simulink model "UDE"  (R2020b)
settings: Solver=VariableStepAuto  StartTime=0.0  StopTime=10.0  RelTol=1e-3
settings Model: Creator=ashya  LastModifiedBy=ashya

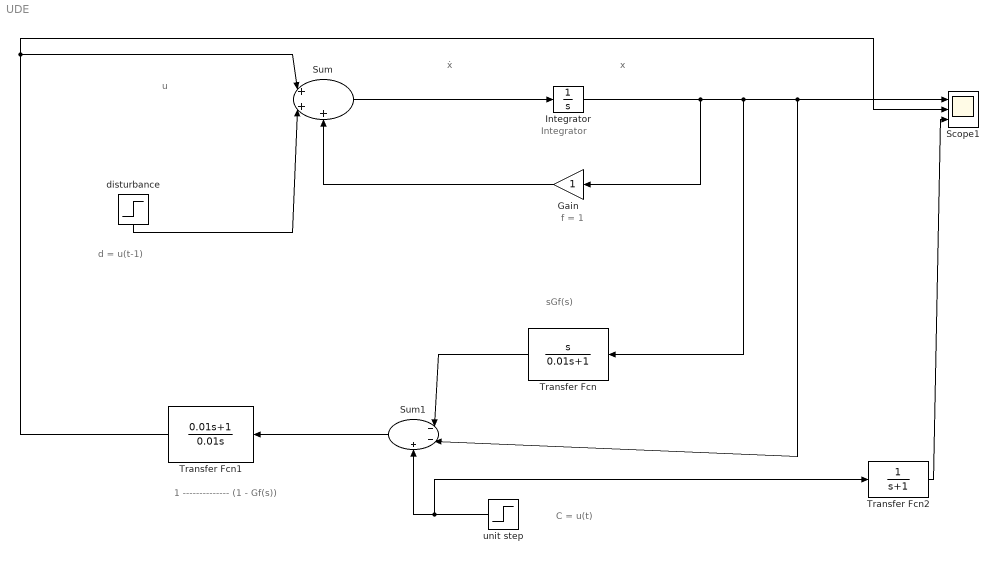
== system UDE ==
  note: sGf(s)
  note: 1
      | --------------
      | (1 - Gf(s))
  note: Integrator
  note: x
  note: ẋ
  note: C = u(t)
  note: f = 1
  note: d = u(t-1)
  note: u
  Gain : Gain
  Integrator : Integrator
  Scope1 : Scope  NumInputPorts=3
  Sum : Sum  Inputs=|+++
  Sum1 : Sum  Inputs=|--+
  Transfer Fcn : TransferFcn  Numerator=[1 0]  Denominator=[0.01 1]
  Transfer Fcn1 : TransferFcn  Numerator=[0.01 1]  Denominator=[0.01 0]
  Transfer Fcn2 : TransferFcn  Denominator=[1 1]
  disturbance : Step  SampleTime=0
  unit step : Step  Time=0  SampleTime=0
  wires:
  Integrator/1 -> Gain/1, Transfer Fcn/1, Sum1/2, Scope1/1
  Sum/1 -> Integrator/1
  Gain/1 -> Sum/3
  disturbance/1 -> Sum/2
  unit step/1 -> Transfer Fcn2/1, Sum1/3
  Transfer Fcn/1 -> Sum1/1
  Sum1/1 -> Transfer Fcn1/1
  Transfer Fcn1/1 -> Scope1/2, Sum/1
  Transfer Fcn2/1 -> Scope1/3
